simulink model "Filter_Design"  (R2020a)
settings: Solver=VariableStepAuto  StartTime=0.0  StopTime=10.0  RelTol=1e-3
settings Model: Creator=Viraj  LastModifiedBy=Viraj

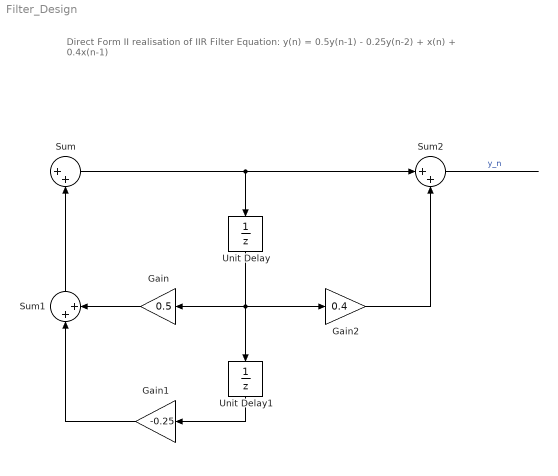
== system Filter_Design ==
  note: Direct Form II realisation of IIR Filter
      |
      | Equation:
      | y(n) = 0.5y(n-1) - 0.25y(n-2) + x(n) + 0.4x(n-1)
  Gain : Gain  Gain=0.5
  Gain1 : Gain  Gain=-0.25
  Gain2 : Gain  Gain=0.4
  Sum : Sum  Inputs=|++
  Sum1 : Sum  Inputs=|++
  Sum2 : Sum  Inputs=|++
  Unit Delay : UnitDelay  SampleTime=-1  HasFrameUpgradeWarning=on
  Unit Delay1 : UnitDelay  SampleTime=-1  HasFrameUpgradeWarning=on
  wires:
  Sum/1 -> Unit Delay/1, Sum2/1
  Unit Delay/1 -> Gain2/1, Gain/1, Unit Delay1/1
  Unit Delay1/1 -> Gain1/1
  Sum1/1 -> Sum/2
  Gain/1 -> Sum1/2
  Gain1/1 -> Sum1/1
  Gain2/1 -> Sum2/2
  ? -> Sum/1  "x_n"
  Sum2/1 -> ?  "y_n"
